simulink model "projeto"  (R2013a)
settings: Solver=ode45  StartTime=0.0  StopTime=10  RelTol=1e-3
values from neighbouring files (symbols this model uses):
  d = 0.6    [controladores.m]
  Ftri = 1e3    (= 1000)    [controladores.m]
  g = 9.81    [controladores.m]
  I = m*d*d/3    (= 0.48)    [controladores.m]
  J = 2.22e-2    (= 0.0222)    [controladores.m]
  k = k(1)    [controladores.m]
  La = 28e-3    (= 0.028)    [controladores.m]
  m = 4    [controladores.m]
  Ra = 2.58    [controladores.m]
  Tmax = Pn/wmn    (= 20.3454584681)    [controladores.m]
  Vs = 240    [controladores.m]
libraries: powerlib x9, cstblocks x2, simulink x1
settings Model: Creator=Guilherme  LastModifiedBy=Guilherme

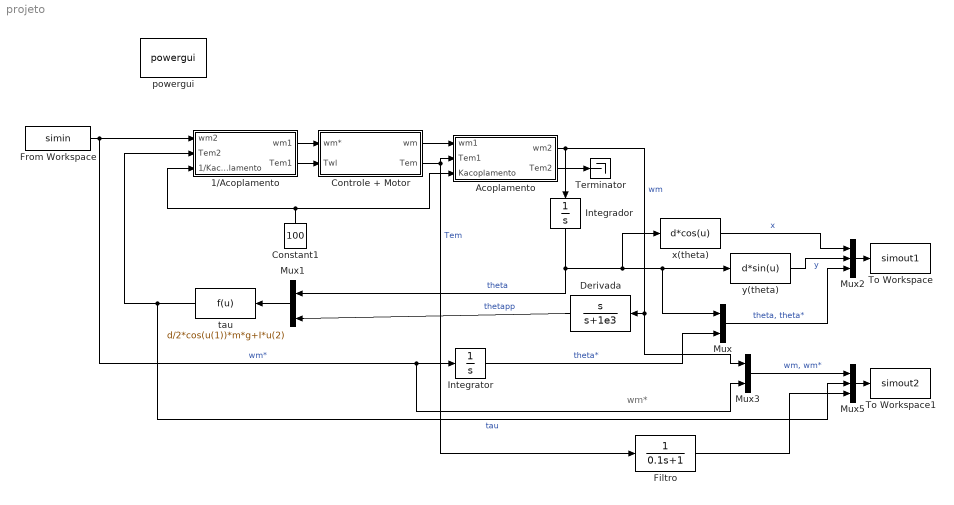
== system projeto ==
  note: wm*
  1/Acoplamento : Subsystem
  Acoplamento : Subsystem
  Constant1 : Constant  Value=100
  Controle + Motor : Subsystem
  Derivada : TransferFcn  Numerator=[1 0]  Denominator=[1 1e3]
  Filtro : TransferFcn  Denominator=[0.1 1]
  From Workspace : FromWorkspace  VariableName=simin  SampleTime=0
  Integrador : Integrator
  Integrator : Integrator
  Mux : Mux  Inputs=2
  Mux1 : Mux  Inputs=2
  Mux2 : Mux  Inputs=3
  Mux3 : Mux  Inputs=2
  Mux5 : Mux  Inputs=3
  Terminator : Terminator
  To Workspace : ToWorkspace  VariableName=simout1  SampleTime=-1  SaveFormat=Timeseries
  To Workspace1 : ToWorkspace  VariableName=simout2  SampleTime=-1  SaveFormat=Timeseries
  powergui : powerlib/powergui  Priority=1  SimulationMode=Discrete  SolverType=Tustin  SampleTime=1e-4  frequency=60  SPID=off  DisableSnubberDevices=off  DisableRonSwitches=off  DisableVfSwitches=off  SwTol=0  Interpol=off  DisplayEquations=off  frequencyindice=0  Pbase=100e6  ErrMax=1e-4  Iterations=50  UnitsV=kV  UnitsW=MW  FunctionMessages=off  echomessages=off  HookPort=off  EnableUseOfTLC=off  x0status=blocks  RestoreLinks=warning  ResistiveCurrentMeasurement=off  Frange=[0:2:500]  Ylog=off  Xlog=on  ShowGrid=off  save=off  variable=ZData  ZoomFFT=off  StartTime=0.0  cycles=1  DisplayStyle=1  fundamental=60  FreqAxis=off  MaxFrequency=1000  frequencyindicesteady=1  RmsSteady=1  display=off  Ts=0  methode=off
  tau : Fcn  Expr=d/2*cos(u(1))*m*g+I*u(2)
  x(theta) : Fcn  Expr=d*cos(u)
  y(theta) : Fcn  Expr=d*sin(u)
  wires:
  Constant1/1 -> Acoplamento/3(Kacoplamento), 1/Acoplamento/3(1/Kacoplamento)
  From Workspace/1 -> 1/Acoplamento/1(wm2), Mux3/2, Integrator/1  "wm*"
  1/Acoplamento/1(wm1) -> Controle + Motor/1(wm*)
  1/Acoplamento/2(Tem1) -> Controle + Motor/2(Twl)
  Controle + Motor/1(wm) -> Acoplamento/1(wm1)
  Integrador/1 -> Mux1/1, x(theta)/1, Mux/1, y(theta)/1  "theta"
  tau/1 -> Mux5/2, 1/Acoplamento/2(Tem2)  "tau"
  Mux1/1 -> tau/1
  Derivada/1 -> Mux1/2  "thetapp"
  x(theta)/1 -> Mux2/1  "x"
  y(theta)/1 -> Mux2/2  "y"
  Mux/1 -> Mux2/3  "theta, theta*"
  Integrator/1 -> Mux/2  "theta*"
  Mux2/1 -> To Workspace/1
  Mux5/1 -> To Workspace1/1
  Mux3/1 -> Mux5/1  "wm, wm*"
  Acoplamento/1(wm2) -> Mux3/1, Derivada/1, Integrador/1  "wm"
  Controle + Motor/2(Tem) -> Acoplamento/2(Tem1), Filtro/1  "Tem"
  Acoplamento/2(Tem2) -> Terminator/1
  Filtro/1 -> Mux5/3

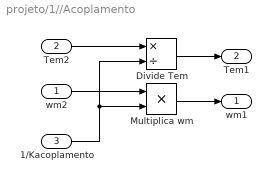
== system projeto/1//Acoplamento ==
  wm2 : Inport
  Tem2 : Inport  Port=2
  1/Kacoplamento : Inport  Port=3
  Divide Tem : Product  Inputs=*/
  Multiplica wm : Product  Inputs=**
  wm1 : Outport
  Tem1 : Outport  Port=2
  wires:
  Tem2/1 -> Divide Tem/1
  1/Kacoplamento/1 -> Multiplica wm/2, Divide Tem/2
  wm2/1 -> Multiplica wm/1
  Multiplica wm/1 -> wm1/1
  Divide Tem/1 -> Tem1/1

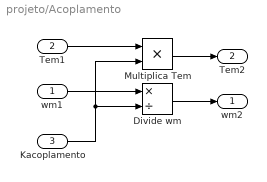
== system projeto/Acoplamento ==
  wm1 : Inport
  Tem1 : Inport  Port=2
  Kacoplamento : Inport  Port=3
  Divide wm : Product  Inputs=*/
  Multiplica Tem : Product  Inputs=**
  wm2 : Outport
  Tem2 : Outport  Port=2
  wires:
  Tem1/1 -> Multiplica Tem/1
  Kacoplamento/1 -> Divide wm/2, Multiplica Tem/2
  wm1/1 -> Divide wm/1
  Divide wm/1 -> wm2/1
  Multiplica Tem/1 -> Tem2/1

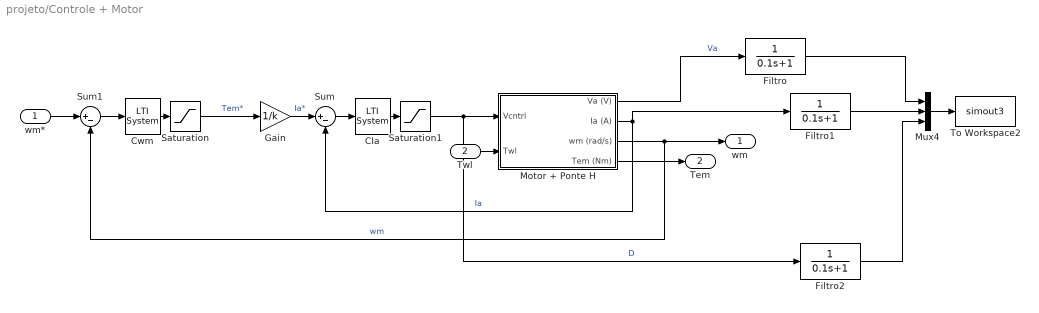
== system projeto/Controle + Motor ==
  wm* : Inport
  Twl : Inport  Port=2
  CIa : cstblocks/LTI System  sys=CIa  IC=[]
  Cwm : cstblocks/LTI System  sys=Cwm  IC=[]
  Filtro : TransferFcn  Denominator=[0.1 1]
  Filtro1 : TransferFcn  Denominator=[0.1 1]
  Filtro2 : TransferFcn  Denominator=[0.1 1]
  Gain : Gain  Gain=1/k
  Motor + Ponte H : Subsystem
  Mux4 : Mux  Inputs=3
  Saturation : Saturate  UpperLimit=Tmax  LowerLimit=-Tmax
  Saturation1 : Saturate  UpperLimit=1  LowerLimit=-1
  Sum : Sum  Inputs=|+-
  Sum1 : Sum  Inputs=|+-
  To Workspace2 : ToWorkspace  VariableName=simout3  SampleTime=-1  SaveFormat=Timeseries
  wm : Outport
  Tem : Outport  Port=2
  wires:
  Twl/1 -> Motor + Ponte H/2(Twl)
  Motor + Ponte H/2(Ia (A)) -> Sum/2, Filtro1/1  "Ia"
  Sum/1 -> CIa/1
  Sum1/1 -> Cwm/1
  Motor + Ponte H/3(wm (rad/s)) -> wm/1, Sum1/2  "wm"
  Cwm/1 -> Saturation/1
  Gain/1 -> Sum/1  "Ia*"
  wm*/1 -> Sum1/1
  Saturation/1 -> Gain/1  "Tem*"
  CIa/1 -> Saturation1/1
  Saturation1/1 -> Filtro2/1, Motor + Ponte H/1(Vcntrl)  "D"
  Motor + Ponte H/4(Tem (Nm)) -> Tem/1
  Motor + Ponte H/1(Va (V)) -> Filtro/1  "Va"
  Mux4/1 -> To Workspace2/1
  Filtro/1 -> Mux4/1
  Filtro1/1 -> Mux4/2
  Filtro2/1 -> Mux4/3

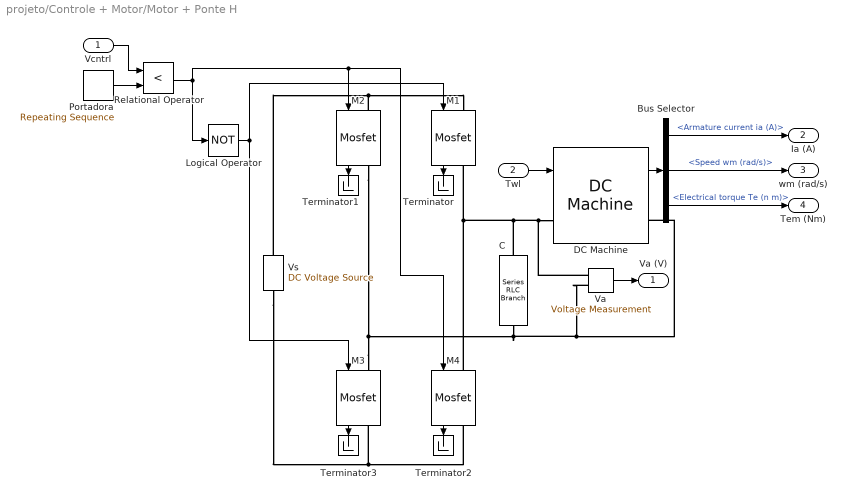
== system projeto/Controle + Motor/Motor + Ponte H ==
  Vcntrl : Inport
  Twl : Inport  Port=2
  Bus Selector : BusSelector  OutputSignals=Armature current ia (A),Speed wm (rad/s),Electrical torque Te (n m)
  C : powerlib/Elements/Series RLC Branch  LConnTagsString=__new0  RConnTagsString=__new0  BranchType=C  Resistance=1  Inductance=1e-3  SetiL0=off  InitialCurrent=0  Capacitance=0.1  Setx0=off  InitialVoltage=0  Measurements=None
  DC Machine : powerlib/Machines/DC Machine  PresetModel=No  MechanicalLoad=Torque TL  FieldType=Permanent magnet  ShowDetailedParameters=on  RLa="[ Ra  La ]"  RLf="[ 240  120]"  Laf=1.8  MachineConstant=Torque constant (N.m/A)  Ke=1.8  Kt=k  J=J  Bm=B  Tf=0  w0=1  Ifinit=1  TsPowergui=0  TsBlock=-1
  Logical Operator : Logic  Operator=NOT  AllPortsSameDT=off  OutDataTypeStr=boolean
  M{1..4} (4 alike) : powerlib/Power Electronics/Mosfet  Ron=0.1  Lon=0  Rd=0.01  Vfd=0  IC=0  Rs=1e5  Cs=inf  Measurements=on
  Portadora : simulink/Sources/Repeating Sequence  rep_seq_t=[0 1/(2*Ftri) 1/Ftri]  rep_seq_y=[-1 1 -1]
  Relational Operator : RelationalOperator  Operator=<  OutDataTypeStr=boolean
  Terminator{,1..3} (4 alike) : Terminator
  Va : powerlib/Measurements/Voltage Measurement  PhasorSimulation=off  OutputType=Complex  PSBequivalent=0
  Vs : powerlib/Electrical Sources/DC Voltage Source  Amplitude=Vs  Measurements=None
  Va (V) : Outport
  Ia (A) : Outport  Port=2
  wm (rad/s) : Outport  Port=3
  Tem (Nm) : Outport  Port=4
  wires:
  Twl/1 -> DC Machine/1
  DC Machine/1 -> Bus Selector/1
  Portadora/1 -> Relational Operator/2
  Relational Operator/1 -> M4/1, M2/1, Logical Operator/1
  Logical Operator/1 -> M3/1, M1/1
  Vcntrl/1 -> Relational Operator/1
  Va/1 -> Va (V)/1
  Bus Selector/2 -> wm (rad/s)/1  "<Speed wm (rad/s)>"
  Bus Selector/1 -> Ia (A)/1  "<Armature current ia (A)>"
  Bus Selector/3 -> Tem (Nm)/1  "<Electrical torque Te (n m)>"
  M1/1 -> Terminator/1
  M2/1 -> Terminator1/1
  M4/1 -> Terminator2/1
  M3/1 -> Terminator3/1
  connections:
  M3/LConn1 -- M2/RConn1 -- Va/LConn2 -- DC Machine/RConn1 -- C/LConn1
  DC Machine/LConn1 -- M1/RConn1 -- M4/LConn1 -- C/RConn1 -- Va/LConn1
  Vs/RConn1 -- M2/LConn1 -- M1/LConn1
  Vs/LConn1 -- M3/RConn1 -- M4/RConn1
